simulink model "HW01_con2"  (R2020a)
settings: Solver=VariableStepAuto  StartTime=0.0  StopTime=10.0  RelTol=1e-3
undefined symbols (not defined in the file or in its folder): par
libraries: simulink x3, Delft_Tyre_dtlib x1, Delft_Tyre_sm1glib x1
settings Model: Creator=Linxi Ren  LastModifiedBy=Linxi Ren
settings DebuggingCC: UnconnectedInputMsg=none  UnconnectedOutputMsg=none  UnconnectedLineMsg=none  SFMachineParentedDataDiag=error

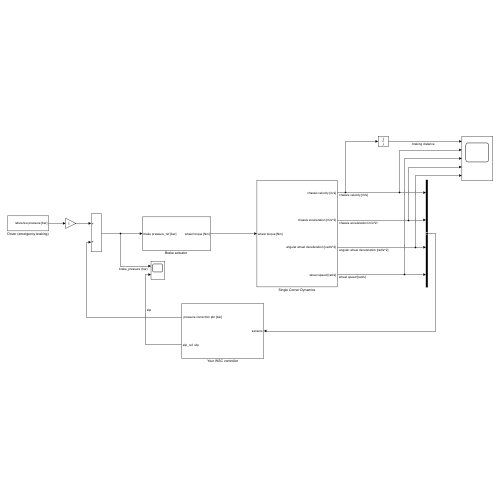
[thumbnail: Simulink's stored preview of the top-level diagram]
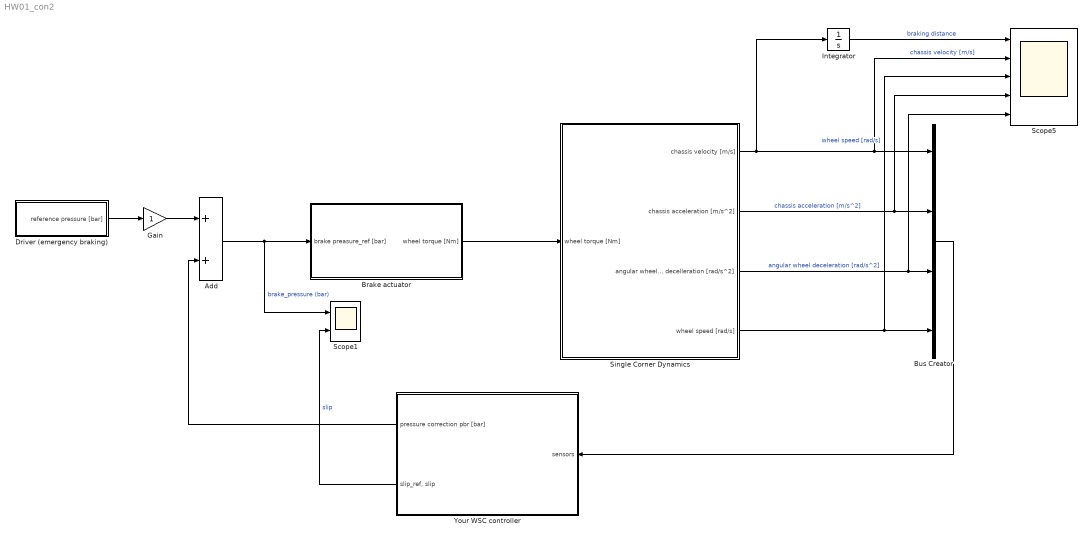
== system HW01_con2 ==
  Add : Sum
  "Brake actuator " : Subsystem
  Bus Creator : BusCreator  Inputs=4
  Driver (emergency braking) : Subsystem
  Gain : Gain
  Integrator : Integrator
  Scope1 : Scope  NumInputPorts=2
  Scope5 : Scope  NumInputPorts=5
  Single Corner Dynamics : Subsystem
  Your WSC controller : Subsystem
  wires:
  Single Corner Dynamics/1(chassis velocity [m/s]) -> Integrator/1, Scope5/2, Bus Creator/1  "chassis velocity [m/s]"
  Your WSC controller/2("slip_ref, slip") -> Scope1/2  "slip"
  Single Corner Dynamics/2(chassis acceleration [m/s^2]) -> Bus Creator/2, Scope5/4  "chassis acceleration [m/s^2]"
  Gain/1 -> Add/1
  Your WSC controller/1(" pressure correction pbr [bar]") -> Add/2
  "Brake actuator "/1(wheel torque [Nm]) -> Single Corner Dynamics/1(wheel torque [Nm])
  Single Corner Dynamics/4(wheel speed [rad/s]) -> Bus Creator/4, Scope5/3  "wheel speed [rad/s]"
  Single Corner Dynamics/3(angular wheel decelleration [rad/s^2]) -> Scope5/5, Bus Creator/3  "angular wheel deceleration [rad/s^2]"
  Bus Creator/1 -> Your WSC controller/1(sensors)
  Integrator/1 -> Scope5/1  "braking distance"
  Add/1 -> Scope1/1, "Brake actuator "/1(brake preasure_ref [bar])  "brake_pressure (bar)"
  Driver (emergency braking)/1(reference pressure [bar]) -> Gain/1

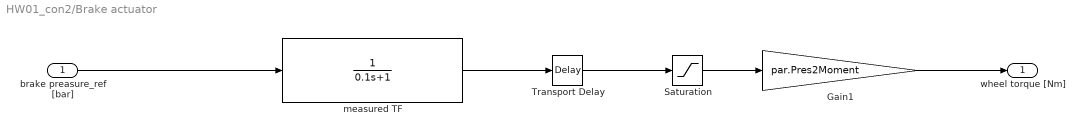
== system HW01_con2/Brake actuator  ==
  brake preasure_ref [bar] : Inport
  " measured TF " : TransferFcn  Denominator=[0.1 1]
  Gain1 : Gain  Gain=par.Pres2Moment
  Saturation : Saturate  UpperLimit=par.max_pressure  LowerLimit=0
  Transport Delay : TransportDelay  DelayTime=0.06
  wheel torque [Nm] : Outport  VectorParamsAs1DForOutWhenUnconnected=off
  wires:
  Gain1/1 -> wheel torque [Nm]/1
  " measured TF "/1 -> Transport Delay/1
  Transport Delay/1 -> Saturation/1
  Saturation/1 -> Gain1/1
  brake preasure_ref [bar]/1 -> " measured TF "/1

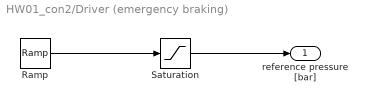
== system HW01_con2/Driver (emergency braking) ==
  Ramp : simulink/Sources/Ramp  slope=100  start=2  InitialOutput=0
  Saturation : Saturate  UpperLimit=100  LowerLimit=0
  reference pressure [bar] : Outport  VectorParamsAs1DForOutWhenUnconnected=off
  wires:
  Ramp/1 -> Saturation/1
  Saturation/1 -> reference pressure [bar]/1

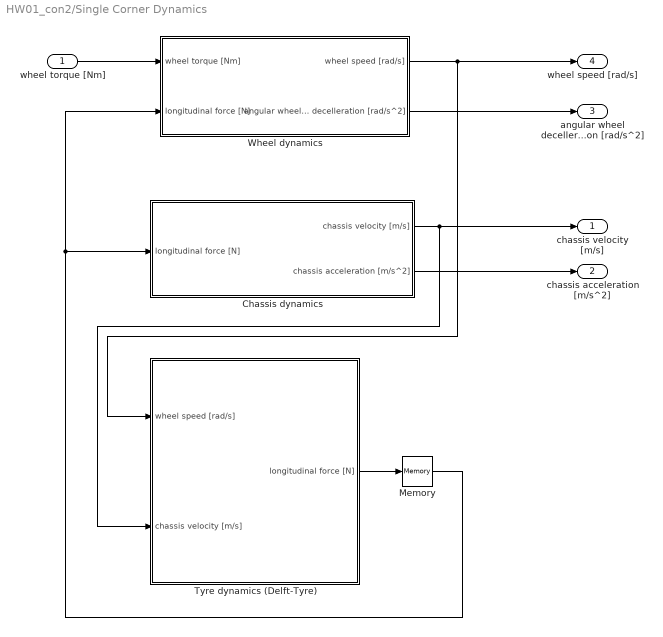
== system HW01_con2/Single Corner Dynamics ==
  wheel torque [Nm] : Inport
  Chassis dynamics : Subsystem
  Memory : Memory
  Tyre dynamics (Delft-Tyre) : Subsystem
  Wheel dynamics : Subsystem
  chassis velocity [m/s] : Outport  VectorParamsAs1DForOutWhenUnconnected=off
  chassis acceleration [m/s^2] : Outport  Port=2  VectorParamsAs1DForOutWhenUnconnected=off
  angular wheel decelleration [rad/s^2] : Outport  Port=3  VectorParamsAs1DForOutWhenUnconnected=off
  wheel speed [rad/s] : Outport  Port=4  VectorParamsAs1DForOutWhenUnconnected=off
  wires:
  wheel torque [Nm]/1 -> Wheel dynamics/1(wheel torque [Nm])
  Wheel dynamics/1(wheel speed [rad/s]) -> Tyre dynamics (Delft-Tyre)/1(wheel speed [rad/s]), wheel speed [rad/s]/1
  Chassis dynamics/1(chassis velocity [m/s]) -> Tyre dynamics (Delft-Tyre)/2(chassis velocity [m/s]), chassis velocity [m/s]/1
  Tyre dynamics (Delft-Tyre)/1(longitudinal force [N]) -> Memory/1
  Memory/1 -> Wheel dynamics/2(longitudinal force [N]), Chassis dynamics/1(longitudinal force [N])
  Wheel dynamics/2(angular wheel decelleration [rad/s^2]) -> angular wheel decelleration [rad/s^2]/1
  Chassis dynamics/2(chassis acceleration [m/s^2]) -> chassis acceleration [m/s^2]/1

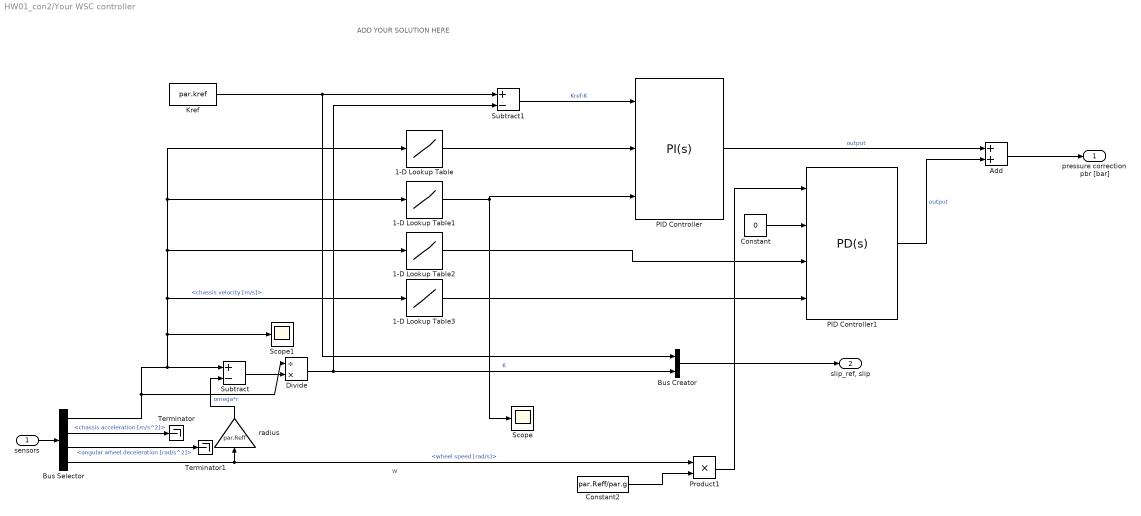
== system HW01_con2/Your WSC controller ==
  note: w
  note: ADD YOUR SOLUTION HERE
  sensors : Inport
  1-D Lookup Table : Lookup_n-D  NumberOfTableDimensions=1  BreakpointsForDimension1=[3;5;15;25;30]  Table=[0;30*1.1;40*1.2;50*1.1;50*0.9]  InternalRulePriority=Speed  RndMeth=Simplest  InputSameDT=on
  1-D Lookup Table1 : Lookup_n-D  NumberOfTableDimensions=1  BreakpointsForDimension1=[0;5;15;25;30]  Table=[3000*3;3000*1.8;3000*1.8;3000*1.5;3000*1.5]  InternalRulePriority=Speed  RndMeth=Simplest  InputSameDT=on
  1-D Lookup Table2 : Lookup_n-D  NumberOfTableDimensions=1  BreakpointsForDimension1=[0;5;15;25;30]  Table=[40;50;50;55;55]  InternalRulePriority=Speed  RndMeth=Simplest  InputSameDT=on
  1-D Lookup Table3 : Lookup_n-D  NumberOfTableDimensions=1  BreakpointsForDimension1=[0;5;15;25;30]  Table=[100;100;100;100;100]  InternalRulePriority=Speed  RndMeth=Simplest  InputSameDT=on
  Add : Sum
  Bus Creator : BusCreator  Inputs=2
  Bus Selector : BusSelector  OutputSignals=chassis velocity [m/s],chassis acceleration [m/s^2],angular wheel deceleration [rad/s^2],wheel speed [rad/s]
  Constant : Constant  Value=0
  Constant2 : Constant  Value=par.Reff/par.g
  Divide : Product  Inputs=/*
  Kref : Constant  Value=par.kref
  PID Controller : simulink/Continuous/PID Controller  Controller=PI  Form=Parallel  TimeDomain=Continuous-time  UseExternalTs=off  SampleTime=-1  IntegratorMethod=Forward Euler  ControllerParametersSource=external  P=115*0.95  I=75*0.95  D=1*0.8  N=100  UseFilter=on  TunerSelectOption=Transfer Function Based (PID Tuner App)  InitialConditionSource=internal  InitialConditionForIntegrator=0  InitialConditionForFilter=0  DifferentiatorICPrevScaledInput=0  ExternalReset=none  TrackingMode=off  Kt=1  LimitOutput=off  UpperSaturationLimit=inf  LowerSaturationLimit=-inf  LinearizeAsGain=on  AntiWindupMode=clamping  Kb=1  POutMin=[]  POutMax=[]  IOutMin=[]  IOutMax=[]  DOutMin=[]  DOutMax=[]  NOutMin=[]  NOutMax=[]  SumOutMin=[]  SumOutMax=[]  SaturationOutMin=[]  SaturationOutMax=[]  PParamMin=[]  PParamMax=[]  IParamMin=[]  IParamMax=[]  DParamMin=[]  DParamMax=[]  NParamMin=[]  NParamMax=[]  KbParamMin=[]  KbParamMax=[]  KtParamMin=[]  KtParamMax=[]  KbOutMin=[]  KbOutMax=[]  KtOutMin=[]  KtOutMax=[]  IntegratorOutMin=[]  IntegratorOutMax=[]  FilterOutMin=[]  FilterOutMax=[]  SumI1OutMin=[]  SumI1OutMax=[]  SumI2OutMin=[]  SumI2OutMax=[]  SumI3OutMin=[]  SumI3OutMax=[]  SumI4OutMin=[]  SumI4OutMax=[]  SumDOutMin=[]  SumDOutMax=[]  DifferentiatorOutMin=[]  DifferentiatorOutMax=[]  FilterDiffOutCoefMin=[]  FilterDiffOutCoefMax=[]  ReciprocalOutMin=[]  ReciprocalOutMax=[]  SumDenOutMin=[]  SumDenOutMax=[]  SumNumOutMin=[]  SumNumOutMax=[]  DivideOutMin=[]  DivideOutMax=[]  UdiffTsProdOutMin=[]  UdiffTsProdOutMax=[]  NTsProdOutMin=[]  NTsProdOutMax=[]  UintegralTsProdOutMin=[]  UintegralTsProdOutMax=[]  UngainTsProdOutMin=[]  UngainTsProdOutMax=[]  IntegratorContinuousStateAttributes=''  IntegratorStateMustResolveToSignalObject=off  IntegratorRTWStateStorageClass=Auto  FilterContinuousStateAttributes=''  FilterStateMustResolveToSignalObject=off  FilterRTWStateStorageClass=Auto  ParallelPVariant=ExternalParameters  IdealPVariant=Disabled  IVariant=ExternalParameters  DVariant=Disabled  IntegratorVariant=Continuous  SatVariant=Disabled  AWVariant=Passthrough  PCopyVariant=Disabled  TRVariant=Disabled  FdbkBlocksVariant=Forward  IdealPFdbkVariant=Disabled  SatFdbkVariant=Disabled  DerivativeFilterVariant=Disabled  NVariant=Disabled  NCopyVariant=Disabled_SignalSpec  FilterICVariant=Disabled  IntegratorICVariant=InternalICs  ExternalResetVariant=Disabled  TRSumVariant=Passthrough  SumFdbkVariant=Disabled  SumVariant=Sum_PI  TsampFilterVariant=InternalTs  TsampNgainVariant=Passthrough  TsampIntegralVariant=Passthrough
  PID Controller1 : simulink/Continuous/PID Controller  Controller=PD  Form=Parallel  TimeDomain=Continuous-time  UseExternalTs=off  SampleTime=-1  IntegratorMethod=Forward Euler  ControllerParametersSource=external  P=115*0.95  I=75*0.95  D=1*0.8  N=100  UseFilter=on  TunerSelectOption=Transfer Function Based (PID Tuner App)  InitialConditionSource=internal  InitialConditionForIntegrator=0  InitialConditionForFilter=0  DifferentiatorICPrevScaledInput=0  ExternalReset=none  TrackingMode=off  Kt=1  LimitOutput=off  UpperSaturationLimit=inf  LowerSaturationLimit=-inf  LinearizeAsGain=on  AntiWindupMode=clamping  Kb=1  POutMin=[]  POutMax=[]  IOutMin=[]  IOutMax=[]  DOutMin=[]  DOutMax=[]  NOutMin=[]  NOutMax=[]  SumOutMin=[]  SumOutMax=[]  SaturationOutMin=[]  SaturationOutMax=[]  PParamMin=[]  PParamMax=[]  IParamMin=[]  IParamMax=[]  DParamMin=[]  DParamMax=[]  NParamMin=[]  NParamMax=[]  KbParamMin=[]  KbParamMax=[]  KtParamMin=[]  KtParamMax=[]  KbOutMin=[]  KbOutMax=[]  KtOutMin=[]  KtOutMax=[]  IntegratorOutMin=[]  IntegratorOutMax=[]  FilterOutMin=[]  FilterOutMax=[]  SumI1OutMin=[]  SumI1OutMax=[]  SumI2OutMin=[]  SumI2OutMax=[]  SumI3OutMin=[]  SumI3OutMax=[]  SumI4OutMin=[]  SumI4OutMax=[]  SumDOutMin=[]  SumDOutMax=[]  DifferentiatorOutMin=[]  DifferentiatorOutMax=[]  FilterDiffOutCoefMin=[]  FilterDiffOutCoefMax=[]  ReciprocalOutMin=[]  ReciprocalOutMax=[]  SumDenOutMin=[]  SumDenOutMax=[]  SumNumOutMin=[]  SumNumOutMax=[]  DivideOutMin=[]  DivideOutMax=[]  UdiffTsProdOutMin=[]  UdiffTsProdOutMax=[]  NTsProdOutMin=[]  NTsProdOutMax=[]  UintegralTsProdOutMin=[]  UintegralTsProdOutMax=[]  UngainTsProdOutMin=[]  UngainTsProdOutMax=[]  IntegratorContinuousStateAttributes=''  IntegratorStateMustResolveToSignalObject=off  IntegratorRTWStateStorageClass=Auto  FilterContinuousStateAttributes=''  FilterStateMustResolveToSignalObject=off  FilterRTWStateStorageClass=Auto  ParallelPVariant=ExternalParameters  IdealPVariant=Disabled  IVariant=Disabled  DVariant=ExternalParameters  IntegratorVariant=Disabled  SatVariant=Disabled  AWVariant=Disabled  PCopyVariant=Disabled  TRVariant=Disabled  FdbkBlocksVariant=Forward  IdealPFdbkVariant=Disabled  SatFdbkVariant=Disabled  DerivativeFilterVariant=ContFilter  NVariant=ExternalParameters  NCopyVariant=Disabled  FilterICVariant=InternalICsFilter  IntegratorICVariant=Disabled  ExternalResetVariant=Disabled  TRSumVariant=Passthrough  SumFdbkVariant=Disabled  SumVariant=Sum_PD  TsampFilterVariant=InternalTs  TsampNgainVariant=Passthrough  TsampIntegralVariant=Disabled_SignalSpec
  Product1 : Product
  Scope : Scope
  Scope1 : Scope
  Subtract : Sum  Inputs=+-
  Subtract1 : Sum  Inputs=+-
  Terminator : Terminator
  Terminator1 : Terminator
  radius : Gain  Gain=par.Reff
  " pressure correction pbr [bar]" : Outport  VectorParamsAs1DForOutWhenUnconnected=off
  "slip_ref, slip" : Outport  Port=2
  wires:
  sensors/1 -> Bus Selector/1
  Bus Selector/3 -> Terminator1/1  "<angular wheel deceleration [rad/s^2]>"
  Bus Selector/2 -> Terminator/1  "<chassis acceleration [m/s^2]>"
  Bus Selector/1 -> Scope1/1, 1-D Lookup Table/1, 1-D Lookup Table1/1, 1-D Lookup Table2/1, 1-D Lookup Table3/1, Subtract/1, Divide/1  "<chassis velocity [m/s]>"
  Subtract/1 -> Divide/2
  Kref/1 -> Subtract1/1, Bus Creator/1
  Divide/1 -> Bus Creator/2, Subtract1/2  "K"
  Bus Selector/4 -> radius/1, Product1/1  "<wheel speed [rad/s]>"
  radius/1 -> Subtract/2  "omega*r"
  Subtract1/1 -> PID Controller/1  "Kref-K"
  PID Controller/1 -> Add/1  "output"
  Bus Creator/1 -> "slip_ref, slip"/1
  1-D Lookup Table/1 -> PID Controller/2
  1-D Lookup Table2/1 -> PID Controller1/3
  1-D Lookup Table3/1 -> PID Controller1/4
  Constant/1 -> PID Controller1/2
  PID Controller1/1 -> Add/2  "output"
  Add/1 -> " pressure correction pbr [bar]"/1
  Constant2/1 -> Product1/2
  Product1/1 -> PID Controller1/1
  1-D Lookup Table1/1 -> PID Controller/3, Scope/1

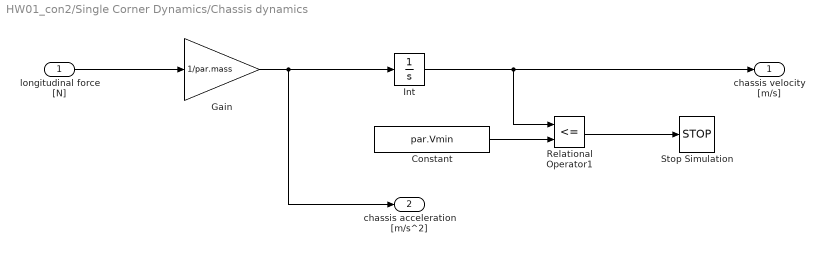
== system HW01_con2/Single Corner Dynamics/Chassis dynamics ==
  longitudinal force [N] : Inport
  Constant : Constant  Value=par.Vmin
  Gain : Gain  Gain=1/par.mass
  Int : Integrator  InitialCondition=par.V0  LimitOutput=on  UpperSaturationLimit=200/3.6  LowerSaturationLimit=eps
  Relational Operator1 : RelationalOperator  Operator=<=  RndMeth=Nearest  InputSameDT=on
  Stop Simulation : Stop
  chassis velocity [m/s] : Outport  VectorParamsAs1DForOutWhenUnconnected=off
  chassis acceleration [m/s^2] : Outport  Port=2  VectorParamsAs1DForOutWhenUnconnected=off
  wires:
  longitudinal force [N]/1 -> Gain/1
  Int/1 -> Relational Operator1/1, chassis velocity [m/s]/1
  Gain/1 -> chassis acceleration [m/s^2]/1, Int/1
  Relational Operator1/1 -> Stop Simulation/1
  Constant/1 -> Relational Operator1/2

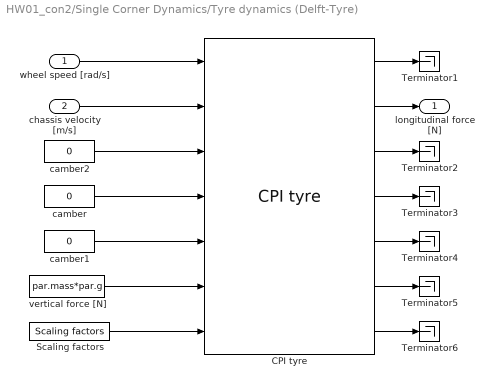
== system HW01_con2/Single Corner Dynamics/Tyre dynamics (Delft-Tyre) ==
  wheel speed [rad/s] : Inport
  chassis velocity [m/s] : Inport  Port=2
  CPI tyre : Delft_Tyre_dtlib/Simulink/CPI tyre  Tag=CPI tyre  idtyre=1  tpfname='TNO_car205_60R15.tir'  side_mode=(3xxx) symmetric  dyn_mode=(xx1x) relaxation behaviour  mf_mode=(xxx1) longitudinal  use_mode=1e8  disp_debug=off
  Scaling factors : Delft_Tyre_sm1glib/SimMechanics 1G/Scaling factors  Tag=Scaling factors  LMUX=par.friction  LKX=1  LMUY=1  LKY=1  LKYC=1  LTR=1  LKZC=1
  Terminator{1..6} (6 alike) : Terminator
  camber : Constant  Value=0
  camber1 : Constant  Value=0
  camber2 : Constant  Value=0
  vertical force [N] : Constant  Value=par.mass*par.g
  longitudinal force [N] : Outport  VectorParamsAs1DForOutWhenUnconnected=off
  wires:
  Scaling factors/1 -> CPI tyre/7
  camber2/1 -> CPI tyre/3
  camber/1 -> CPI tyre/4
  CPI tyre/1 -> Terminator1/1
  CPI tyre/3 -> Terminator2/1
  CPI tyre/4 -> Terminator3/1
  CPI tyre/6 -> Terminator5/1
  CPI tyre/5 -> Terminator4/1
  camber1/1 -> CPI tyre/5
  chassis velocity [m/s]/1 -> CPI tyre/2
  wheel speed [rad/s]/1 -> CPI tyre/1
  CPI tyre/2 -> longitudinal force [N]/1
  vertical force [N]/1 -> CPI tyre/6
  CPI tyre/7 -> Terminator6/1

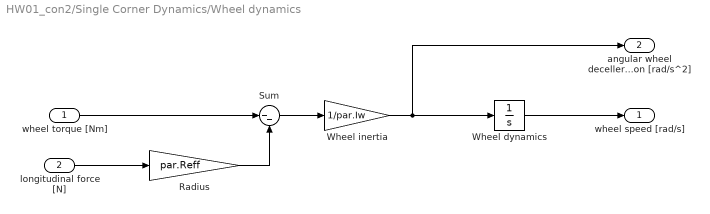
== system HW01_con2/Single Corner Dynamics/Wheel dynamics ==
  wheel torque [Nm] : Inport
  longitudinal force [N] : Inport  Port=2
  Radius : Gain  Gain=par.Reff  SaturateOnIntegerOverflow=on  OutDataTypeStr=Inherit: Same as input  ParamDataTypeStr=Inherit: Same as input
  Sum : Sum  Inputs=|--  InputSameDT=on  SaturateOnIntegerOverflow=on  OutDataTypeStr=Inherit: Same as first input
  Wheel dynamics : Integrator  InitialCondition=par.V0/par.Reff  LimitOutput=on  UpperSaturationLimit=200/3.6/par.Reff  LowerSaturationLimit=eps
  Wheel inertia : Gain  Gain=1/par.Iw  SaturateOnIntegerOverflow=on  OutDataTypeStr=Inherit: Same as input  ParamDataTypeStr=Inherit: Same as input
  wheel speed [rad/s] : Outport  VectorParamsAs1DForOutWhenUnconnected=off
  angular wheel decelleration [rad/s^2] : Outport  Port=2  VectorParamsAs1DForOutWhenUnconnected=off
  wires:
  Wheel inertia/1 -> angular wheel decelleration [rad/s^2]/1, Wheel dynamics/1
  wheel torque [Nm]/1 -> Sum/1
  Wheel dynamics/1 -> wheel speed [rad/s]/1
  Sum/1 -> Wheel inertia/1
  longitudinal force [N]/1 -> Radius/1
  Radius/1 -> Sum/2
